simulink model "double_integrator_sim"  (R2025b)
settings: Solver=VariableStepAuto  StartTime=0.0  StopTime=10.0  RelTol=1e-3
settings Model: Creator=jx2004  LastModifiedBy=jx2004

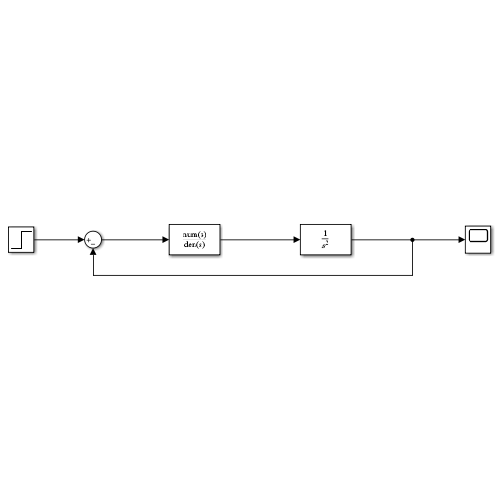
[thumbnail: Simulink's stored preview of the top-level diagram]
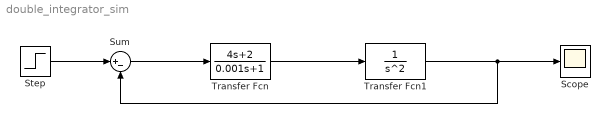
== system double_integrator_sim ==
  Scope : Scope
      settings: ActiveDisplayYMinimum=-0.13535208285686604  ActiveDisplayYMaximum=1.2181687457117945
  Step : Step  SampleTime=0
  Sum : Sum  Inputs=|+-
  Transfer Fcn : TransferFcn  Numerator=[4 2]  Denominator=[0.001 1]
  Transfer Fcn1 : TransferFcn  Denominator=[1 0 0]
  wires:
  Transfer Fcn/1 -> Transfer Fcn1/1
  Sum/1 -> Transfer Fcn/1
  Step/1 -> Sum/1
  Transfer Fcn1/1 -> Sum/2, Scope/1
